simulink model "Problem7"  (R2020a)
settings: Solver=VariableStepAuto  StartTime=0.0  StopTime=10.0  RelTol=1e-3
settings Model: Creator=Shreyas  LastModifiedBy=Shreyas

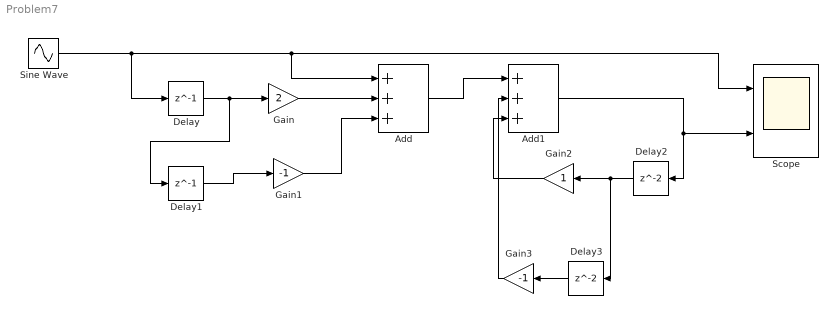
== system Problem7 ==
  Add : Sum  Inputs=+++
  Add1 : Sum  Inputs=+++
  Delay : Delay  DelayLength=1
  Delay1 : Delay  DelayLength=1
  Delay2 : Delay
  Delay3 : Delay
  Gain : Gain  Gain=2
  Gain1 : Gain  Gain=-1
  Gain2 : Gain
  Gain3 : Gain  Gain=-1
  Scope : Scope  NumInputPorts=2
  Sine Wave : Sin  Amplitude=2  SampleTime=0
  wires:
  Sine Wave/1 -> Scope/1, Add/1, Delay/1
  Gain/1 -> Add/2
  Delay/1 -> Delay1/1, Gain/1
  Delay1/1 -> Gain1/1
  Gain1/1 -> Add/3
  Add/1 -> Add1/1
  Gain2/1 -> Add1/3
  Gain3/1 -> Add1/2
  Delay3/1 -> Gain3/1
  Delay2/1 -> Delay3/1, Gain2/1
  Add1/1 -> Scope/2, Delay2/1
